simulink library "GenericTarget"  (R2020b)
settings: Solver=VariableStepAuto  StartTime=0.0  StopTime=10.0  RelTol=1e-3
undefined symbols (not defined in the file or in its folder): CheckUniqueParameterValue
(part 2 of 2)

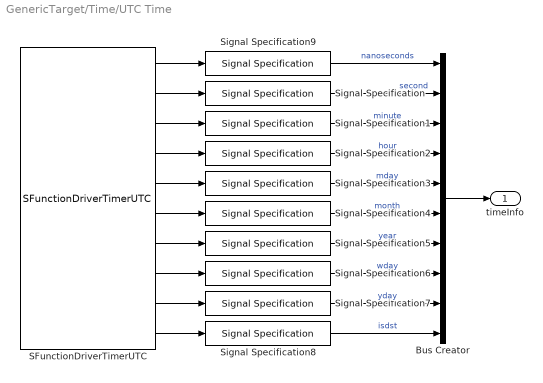
== system GenericTarget/Time/UTC Time ==
  Bus Creator : BusCreator  Inputs=10
  SFunctionDriverTimerUTC : S-Function  FunctionName=SFunctionDriverTimerUTC  Parameters=SampleTime  SFunctionDeploymentMode=off  EnableBusSupport=off  mask(Legacy Function){SFunctionSpec=void OutputDriverTimerUTC(int32 y1[1], int32 y2[1], int32 y3[1], int32 y4[1], int32 y5[1], int32 y6[1], int32 y7[1], int32 y8[1], int32 y9[1], int32 y10[1]), SampleTime=SampleTime, ShowSpec=off}
      mask prompts: SampleTime "Sample time (-1 for inherited):"; ShowSpec "Display function specification"
      mask help:
      | This block allows you to call the legacy functions specified by the following Legacy Code Tool definition:
      | def.SFunctionName = 'SFunctionDriverTimerUTC';
      | def.OutputFcnSpec = 'void OutputDriverTimerUTC(int32 y1[1], int32 y2[1], int32 y3[1], int32 y4[1], int32 y5[1], int32 y6[1], int32 y7[1], int32 y8[1], int32 y9[1], int32 y10[1])';
      | def.StartFcnSpec = 'void CreateDriverTimerUTC()';
      | def.TerminateFcnSpec = 'void DeleteDriverTimerUTC()';
      | def.HeaderFiles = {'DriverTimerUTC.h'};
      | def.SourceFiles = {'DriverTimerUTC.cpp'};
      | def.SampleTime = 'parameterized';
      | def.Options.useTlcWithAccel = false;
      mask Help: <p>This block was generated automatically by the Legacy Code Tool. For detailed help on this tool, call<a href="matlab:legacy_code('help')"> legacy_code('help')</a>.</p>
      mask Callback ShowSpec:
      | if strcmp(get_param(gcbh, 'ShowSpec'), 'on')
      |   set_param(gcbh, 'MaskDisplay', sprintf('fprintf(''%s'');', get_param(gcbh, 'SFunctionSpec')));
      | else
      |   set_param(gcbh, 'MaskDisplay', sprintf('fprintf(''%s'');', get_param(gcbh, 'FunctionName')));
      | end
      mask Display: fprintf('SFunctionDriverTimerUTC');
  Signal Specification : SignalSpecification  OutDataTypeStr=int32  Unit=s  Dimensions=1
  Signal Specification1 : SignalSpecification  OutDataTypeStr=int32  Unit=min  Dimensions=1
  Signal Specification2 : SignalSpecification  OutDataTypeStr=int32  Unit=h  Dimensions=1
  Signal Specification3 : SignalSpecification  OutDataTypeStr=int32  Unit=d  Dimensions=1
  Signal Specification4 : SignalSpecification  OutDataTypeStr=int32  Dimensions=1
  Signal Specification5 : SignalSpecification  OutDataTypeStr=int32  Dimensions=1
  Signal Specification6 : SignalSpecification  OutDataTypeStr=int32  Unit=d  Dimensions=1
  Signal Specification7 : SignalSpecification  OutDataTypeStr=int32  Unit=d  Dimensions=1
  Signal Specification8 : SignalSpecification  OutDataTypeStr=int32  Dimensions=1
  Signal Specification9 : SignalSpecification  OutDataTypeStr=int32  Unit=ns  Dimensions=1
  timeInfo : Outport  VectorParamsAs1DForOutWhenUnconnected=off
  wires:
  Bus Creator/1 -> timeInfo/1
  Signal Specification/1 -> Bus Creator/2  "second"
  Signal Specification1/1 -> Bus Creator/3  "minute"
  Signal Specification2/1 -> Bus Creator/4  "hour"
  Signal Specification3/1 -> Bus Creator/5  "mday"
  Signal Specification4/1 -> Bus Creator/6  "month"
  Signal Specification5/1 -> Bus Creator/7  "year"
  Signal Specification6/1 -> Bus Creator/8  "wday"
  Signal Specification7/1 -> Bus Creator/9  "yday"
  Signal Specification8/1 -> Bus Creator/10  "isdst"
  SFunctionDriverTimerUTC/1 -> Signal Specification9/1
  SFunctionDriverTimerUTC/2 -> Signal Specification/1
  SFunctionDriverTimerUTC/3 -> Signal Specification1/1
  SFunctionDriverTimerUTC/4 -> Signal Specification2/1
  SFunctionDriverTimerUTC/5 -> Signal Specification3/1
  SFunctionDriverTimerUTC/6 -> Signal Specification4/1
  SFunctionDriverTimerUTC/7 -> Signal Specification5/1
  SFunctionDriverTimerUTC/8 -> Signal Specification6/1
  SFunctionDriverTimerUTC/9 -> Signal Specification7/1
  SFunctionDriverTimerUTC/10 -> Signal Specification8/1
  Signal Specification9/1 -> Bus Creator/1  "nanoseconds"

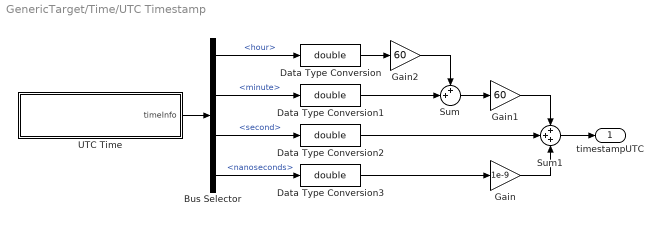
== system GenericTarget/Time/UTC Timestamp ==
  Bus Selector : BusSelector  OutputSignals=hour,minute,second,nanoseconds
  Data Type Conversion{,1..3} (4 alike) : DataTypeConversion  OutDataTypeStr=double
  Gain : Gain  Gain=1e-9
  Gain1 : Gain  Gain=60
  Gain2 : Gain  Gain=60
  Sum : Sum  Inputs=++|
  Sum1 : Sum  Inputs=+++
  UTC Time : Subsystem  mask{SampleTime=SampleTime}
      mask prompts: SampleTime "Sample time (-1 for inherited):"
      mask help:
      | Get the current UTC time of the target. During simulation this block has no effect.<br><br>
      |
      | <b>nanoseconds</b><br>Nanoseconds after the second [0, 999999999].<br><br>
      |
      | <b>second</b><br>Seconds after the minute [0, 60] (60 to allow leap second).<br><br>
      |
      | <b>minute</b><br>Minutes after the hour [0, 59].<br><br>
      |
      | <b>hour</b><br>Hours since midnight [0, 23].<br><br>
      |
      | <b>mday</b><br>Day of the month [1, 31].<br><br>
      |
      | <b>mon</b><br>Month since January [0, 11].<br><br>
      |
      | <b>year</b><br>Years since 1900.<br><br>
      |
      | <b>wday</b><br>Days since Sunday [0, 6].<br><br>
      |
      | <b>yday</b><br>Days since January 1 [0, 365].<br><br>
      |
      | <b>isdst</b><br>Daylight Saving Time flag. The value is positive if DST is in effect, zero if not and negative if no information is available.
      mask DialogControl DescGroupVar Prompt: UTC Time - Generic Target
      mask Display:
      | % Get dimension of block
      | pos = get_param(gcb, 'Position');
      | width = pos(3) - pos(1);
      | height = pos(4) - pos(2);
      | 
      | % Set image to center of block
      | imgSize = 32;
      | image('icon.svg', [0.5*(width-imgSize),0.5*(height-imgSize),imgSize,imgSize]);
      | image('time.svg', [0.5*(height-imgSize),0.5*(height-imgSize),imgSize,imgSize]);
      | 
      | % Set text
      | text(2,2,'UTC','horizontalAlignment','left','verticalAlignment','bottom','texmode','on');
  timestampUTC : Outport  OutDataTypeStr=double  Unit=s  PortDimensions=1  VectorParamsAs1DForOutWhenUnconnected=off
  wires:
  Bus Selector/4 -> Data Type Conversion3/1  "<nanoseconds>"
  Data Type Conversion1/1 -> Sum/2
  UTC Time/1(timeInfo) -> Bus Selector/1
  Data Type Conversion2/1 -> Sum1/2
  Bus Selector/3 -> Data Type Conversion2/1  "<second>"
  Bus Selector/1 -> Data Type Conversion/1  "<hour>"
  Gain1/1 -> Sum1/1
  Data Type Conversion/1 -> Gain2/1
  Gain/1 -> Sum1/3
  Sum1/1 -> timestampUTC/1
  Gain2/1 -> Sum/1
  Bus Selector/2 -> Data Type Conversion1/1  "<minute>"
  Sum/1 -> Gain1/1
  Data Type Conversion3/1 -> Gain/1

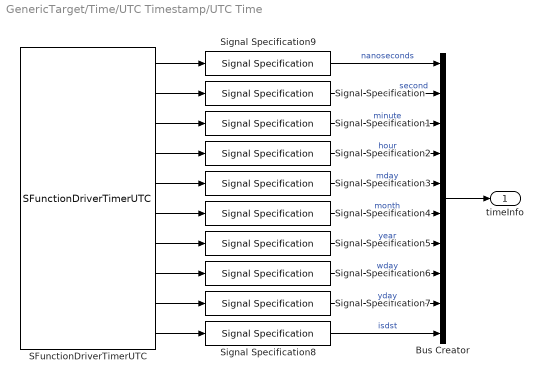
== system GenericTarget/Time/UTC Timestamp/UTC Time ==
  Bus Creator : BusCreator  Inputs=10
  SFunctionDriverTimerUTC : S-Function  FunctionName=SFunctionDriverTimerUTC  Parameters=SampleTime  SFunctionDeploymentMode=off  EnableBusSupport=off  mask(Legacy Function){SFunctionSpec=void OutputDriverTimerUTC(int32 y1[1], int32 y2[1], int32 y3[1], int32 y4[1], int32 y5[1], int32 y6[1], int32 y7[1], int32 y8[1], int32 y9[1], int32 y10[1]), SampleTime=SampleTime, ShowSpec=off}
      mask prompts: SampleTime "Sample time (-1 for inherited):"; ShowSpec "Display function specification"
      mask help:
      | This block allows you to call the legacy functions specified by the following Legacy Code Tool definition:
      | def.SFunctionName = 'SFunctionDriverTimerUTC';
      | def.OutputFcnSpec = 'void OutputDriverTimerUTC(int32 y1[1], int32 y2[1], int32 y3[1], int32 y4[1], int32 y5[1], int32 y6[1], int32 y7[1], int32 y8[1], int32 y9[1], int32 y10[1])';
      | def.StartFcnSpec = 'void CreateDriverTimerUTC()';
      | def.TerminateFcnSpec = 'void DeleteDriverTimerUTC()';
      | def.HeaderFiles = {'DriverTimerUTC.h'};
      | def.SourceFiles = {'DriverTimerUTC.cpp'};
      | def.SampleTime = 'parameterized';
      | def.Options.useTlcWithAccel = false;
      mask Help: <p>This block was generated automatically by the Legacy Code Tool. For detailed help on this tool, call<a href="matlab:legacy_code('help')"> legacy_code('help')</a>.</p>
      mask Callback ShowSpec:
      | if strcmp(get_param(gcbh, 'ShowSpec'), 'on')
      |   set_param(gcbh, 'MaskDisplay', sprintf('fprintf(''%s'');', get_param(gcbh, 'SFunctionSpec')));
      | else
      |   set_param(gcbh, 'MaskDisplay', sprintf('fprintf(''%s'');', get_param(gcbh, 'FunctionName')));
      | end
      mask Display: fprintf('SFunctionDriverTimerUTC');
  Signal Specification : SignalSpecification  OutDataTypeStr=int32  Unit=s  Dimensions=1
  Signal Specification1 : SignalSpecification  OutDataTypeStr=int32  Unit=min  Dimensions=1
  Signal Specification2 : SignalSpecification  OutDataTypeStr=int32  Unit=h  Dimensions=1
  Signal Specification3 : SignalSpecification  OutDataTypeStr=int32  Unit=d  Dimensions=1
  Signal Specification4 : SignalSpecification  OutDataTypeStr=int32  Dimensions=1
  Signal Specification5 : SignalSpecification  OutDataTypeStr=int32  Dimensions=1
  Signal Specification6 : SignalSpecification  OutDataTypeStr=int32  Unit=d  Dimensions=1
  Signal Specification7 : SignalSpecification  OutDataTypeStr=int32  Unit=d  Dimensions=1
  Signal Specification8 : SignalSpecification  OutDataTypeStr=int32  Dimensions=1
  Signal Specification9 : SignalSpecification  OutDataTypeStr=int32  Unit=ns  Dimensions=1
  timeInfo : Outport  VectorParamsAs1DForOutWhenUnconnected=off
  wires:
  Signal Specification9/1 -> Bus Creator/1  "nanoseconds"
  SFunctionDriverTimerUTC/10 -> Signal Specification8/1
  SFunctionDriverTimerUTC/9 -> Signal Specification7/1
  SFunctionDriverTimerUTC/8 -> Signal Specification6/1
  SFunctionDriverTimerUTC/7 -> Signal Specification5/1
  SFunctionDriverTimerUTC/6 -> Signal Specification4/1
  SFunctionDriverTimerUTC/5 -> Signal Specification3/1
  SFunctionDriverTimerUTC/4 -> Signal Specification2/1
  SFunctionDriverTimerUTC/3 -> Signal Specification1/1
  SFunctionDriverTimerUTC/2 -> Signal Specification/1
  SFunctionDriverTimerUTC/1 -> Signal Specification9/1
  Signal Specification8/1 -> Bus Creator/10  "isdst"
  Signal Specification7/1 -> Bus Creator/9  "yday"
  Signal Specification6/1 -> Bus Creator/8  "wday"
  Signal Specification5/1 -> Bus Creator/7  "year"
  Signal Specification4/1 -> Bus Creator/6  "month"
  Signal Specification3/1 -> Bus Creator/5  "mday"
  Signal Specification2/1 -> Bus Creator/4  "hour"
  Signal Specification1/1 -> Bus Creator/3  "minute"
  Signal Specification/1 -> Bus Creator/2  "second"
  Bus Creator/1 -> timeInfo/1
